simulink model "t1_85_withsource"  (R2019b)
settings: Solver=VariableStepAuto  StartTime=0.0  StopTime=0.06  RelTol=1e-3
libraries: powerlib x20, powerlib_meascontrol x2
settings Model: Creator=96547  LastModifiedBy=96547

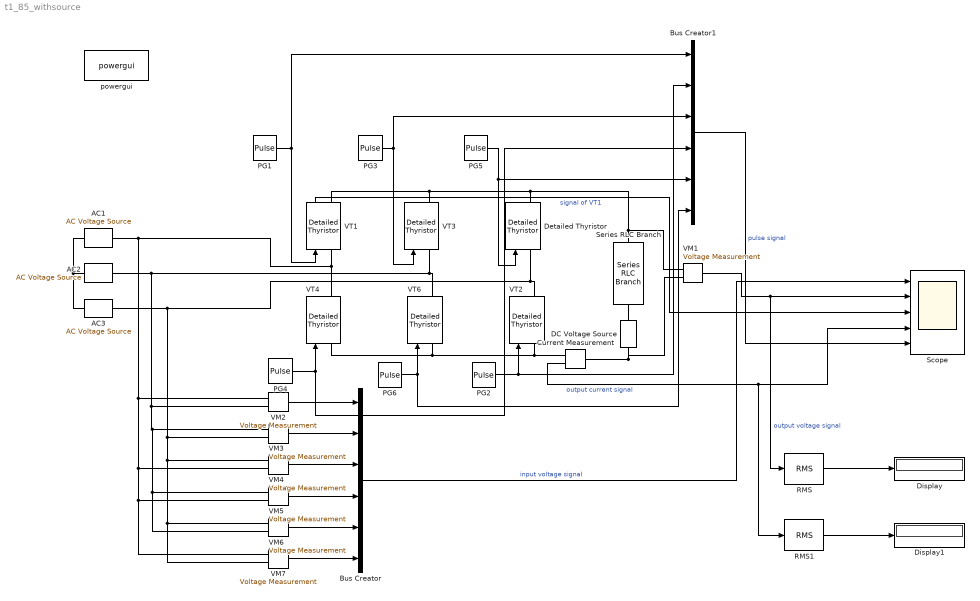
== system t1_85_withsource ==
  AC1 : powerlib/Electrical Sources/AC Voltage Source  Amplitude=220*sqrt(2)  Phase=0  Frequency=50  SampleTime=0  Measurements=None  BusType=swing  Pref=10e3  Qref=0  Qmin=-inf  Qmax=+inf
      settings: SourceProductName=Simscape Electrical
  AC2 : powerlib/Electrical Sources/AC Voltage Source  Amplitude=220*sqrt(2)  Phase=-120  Frequency=50  SampleTime=0  Measurements=Voltage  BusType=swing  Pref=10e3  Qref=0  Qmin=-inf  Qmax=+inf
      settings: SourceProductName=Simscape Electrical
  AC3 : powerlib/Electrical Sources/AC Voltage Source  Amplitude=220*sqrt(2)  Phase=-240  Frequency=50  SampleTime=0  Measurements=None  BusType=swing  Pref=10e3  Qref=0  Qmin=-inf  Qmax=+inf
      settings: SourceProductName=Simscape Electrical
  Bus Creator : BusCreator  Inputs=6
  Bus Creator1 : BusCreator  Inputs=6
  Current Measurement : powerlib/Measurements/Current Measurement  PhasorSimulation=off  OutputType=Complex  PSBequivalent=0
      settings: SourceProductName=Simscape Electrical
  DC Voltage Source : powerlib/Electrical Sources/DC Voltage Source  Amplitude=400  Measurements=None
      settings: SourceProductName=Simscape Electrical
  Detailed Thyristor : powerlib/Power Electronics/Detailed Thyristor  Ron=0.001  Lon=1e-3  Vf=0.8  IL=0.1  Tq=100e-6  IC=0  Rs=500  Cs=250e-9  Measurements=on
      settings: SourceProductName=Simscape Electrical  SourceProductBaseCode=PS
  Display : Display
  Display1 : Display
  PG1 : DiscretePulseGenerator  PulseType=Time based  Amplitude=5  Period=0.02  PulseWidth=20  PhaseDelay=0.0064
  PG2 : DiscretePulseGenerator  PulseType=Time based  Amplitude=5  Period=0.02  PulseWidth=20  PhaseDelay=0.0097
  PG3 : DiscretePulseGenerator  PulseType=Time based  Amplitude=5  Period=0.02  PulseWidth=20  PhaseDelay=0.0131
  PG4 : DiscretePulseGenerator  PulseType=Time based  Amplitude=5  Period=0.02  PulseWidth=20  PhaseDelay=0.0164
  PG5 : DiscretePulseGenerator  PulseType=Time based  Amplitude=5  Period=0.02  PulseWidth=20  PhaseDelay=0.0197
  PG6 : DiscretePulseGenerator  PulseType=Time based  Amplitude=5  Period=0.02  PulseWidth=20  PhaseDelay=0.0231
  RMS : powerlib_meascontrol/Measurements/RMS  TrueRMS=on  Freq=60  RMSInit=120  Ts=0
      settings: SourceProductName=Simscape Electrical
  RMS1 : powerlib_meascontrol/Measurements/RMS  TrueRMS=on  Freq=60  RMSInit=120  Ts=0
      settings: SourceProductName=Simscape Electrical
  Scope : Scope  NumInputPorts=5
  Series RLC Branch : powerlib/Elements/Series RLC Branch  LConnTagsString=__new0  RConnTagsString=__new0  BranchType=RL  Resistance=1  Inductance=5e-3  SetiL0=off  InitialCurrent=0  Capacitance=1e-6  Setx0=off  InitialVoltage=0  Measurements=None
      settings: SourceProductName=Simscape Electrical
  VM{1..7} (7 alike) : powerlib/Measurements/Voltage Measurement  PhasorSimulation=off  OutputType=Complex  PSBequivalent=0
      settings: SourceProductName=Simscape Electrical
  VT{1..4,6} (5 alike) : powerlib/Power Electronics/Detailed Thyristor  Ron=0.001  Lon=1e-3  Vf=0.8  IL=0.1  Tq=100e-6  IC=0  Rs=500  Cs=250e-9  Measurements=on
      settings: SourceProductName=Simscape Electrical  SourceProductBaseCode=PS
  powergui : powerlib/powergui  Priority=1  SimulationMode=Continuous  SampleTime=50e-6  frequency=60  Iterations=50  frequencyindice=50  Pbase=100e6  ErrMax=1e-4  UnitsV=kV  UnitsW=MW  buscounter=0  FunctionMessages=off  echomessages=off  EnableUseOfTLC=off  CurrentSourceSwitches=off  DisableSnubberDevices=off  DisableRonSwitches=off  DisableVfSwitches=off  DisplayEquations=off  AutomaticDiscreteSolvers=off  SolverType=Tustin/Backward Euler (TBE)  Interpol=off  ExternalGateDelay=off  methode=off  Ts=100  x0status=blocks  SPID=on  SwTol=0  HookPort=off  NonlinearTolerance=1e-4  nMaxIteration=100  ContinueOnMaxIteration=off  RestoreLinks=warning  ResistiveCurrentMeasurement=off  Frange=[0:2:500]  Ylog=off  Xlog=on  ShowGrid=off  save=off  variable=ZData  structure=0  ZoomFFT=off  StartTime=0.0  cycles=1  DisplayStyle=1  fundamental=60  FreqAxis=off  MaxFrequency=1000  frequencyindicesteady=1  RmsSteady=1  display=off
      settings: SourceProductName=Simscape Electrical
  wires:
  VM2/1 -> Bus Creator/1
  VM3/1 -> Bus Creator/2
  VM4/1 -> Bus Creator/3
  VM5/1 -> Bus Creator/4
  VM6/1 -> Bus Creator/5
  VM7/1 -> Bus Creator/6
  Bus Creator/1 -> Scope/1  "input voltage signal"
  PG1/1 -> VT1/1, Bus Creator1/1
  PG3/1 -> VT3/1, Bus Creator1/3
  PG5/1 -> Detailed Thyristor/1, Bus Creator1/5
  PG4/1 -> Bus Creator1/4, VT4/1
  PG6/1 -> VT6/1, Bus Creator1/6
  PG2/1 -> VT2/1, Bus Creator1/2
  Current Measurement/1 -> RMS1/1, Scope/4  "output current signal"
  VM1/1 -> RMS/1, Scope/2  "output voltage signal"
  Bus Creator1/1 -> Scope/5  "pulse signal"
  VT1/1 -> Scope/3  "signal of VT1"
  RMS/1 -> Display/1
  RMS1/1 -> Display1/1
  connections:
  VM2/LConn1 -- VM7/LConn1 -- VM5/LConn2 -- VM4/LConn2 -- AC1/RConn1 -- VT1/LConn1 -- VT4/RConn1
  VM1/LConn1 -- Series RLC Branch/LConn1 -- Detailed Thyristor/RConn1 -- VT3/RConn1 -- VT1/RConn1
  VM7/LConn2 -- VM6/LConn1 -- VM4/LConn1 -- VM3/LConn2 -- AC3/RConn1 -- VT2/RConn1 -- Detailed Thyristor/LConn1
  VT2/LConn1 -- Current Measurement/RConn1 -- VT6/LConn1 -- VT4/LConn1
  VM5/LConn1 -- VM6/LConn2 -- VM3/LConn1 -- VM2/LConn2 -- AC2/RConn1 -- VT6/RConn1 -- VT3/LConn1
  AC1/LConn1 -- AC3/LConn1 -- AC2/LConn1
  Current Measurement/LConn1 -- VM1/LConn2 -- DC Voltage Source/LConn1
  Series RLC Branch/RConn1 -- DC Voltage Source/RConn1
